simulink model "test_8m_0508"  (R2024a)
settings: Solver=FixedStepAuto  StartTime=0.0  StopTime=30  FixedStep=dt  RelTol=1e-3
values from neighbouring files (symbols this model uses):
  attitude_0 = [0; -90;  -0]    [ini_param_8m_0522.m]
  b = 4.0    (= 4)    [ini_param_8m_0522.m]
  cbar = 0.75    [ini_param_8m_0522.m]
  dt = 0.004    [ini_param_8m_0522.m]
  H = 1000    [ini_param_8m_0522.m]
  N_data = [0,200, 491, 804, 1077, 1344, 1559, 1832, 2078, 2318, 2579,            2864, 3117, 3371, 3608.2, 3872, 4055.7, 4291, 4507, 4739, 4935]'    [cal_motor.m]
  N_pwm = 0.01*[0, 5 ,10 ,15 ,20 ,25 ,30 ,35,40, 45 ,50 ,              55 ,60 ,65 ,70, 75, 80 , 85 ,90 ,95 ,100]'    [cal_motor.m]
  pitch_rate_K = 1    [ini_param_8m_0522.m]
  roll_rate_K = 1    [ini_param_8m_0522.m]
  S = 6.0    (= 6)    [ini_param_8m_0522.m]
  Ts = 0.05    [ini_param_8m_0522.m]
  Ts_sur = 0.25    [ini_param_8m_0522.m]
  yaw_rate_K = 1    [ini_param_8m_0522.m]
undefined symbols (not defined in the file or in its folder): sigbuilder_block, UAV
libraries: slpidlib x9, simulink_extras x6, sharedtransform x2, shared6dof x1
(part 11 of 11)

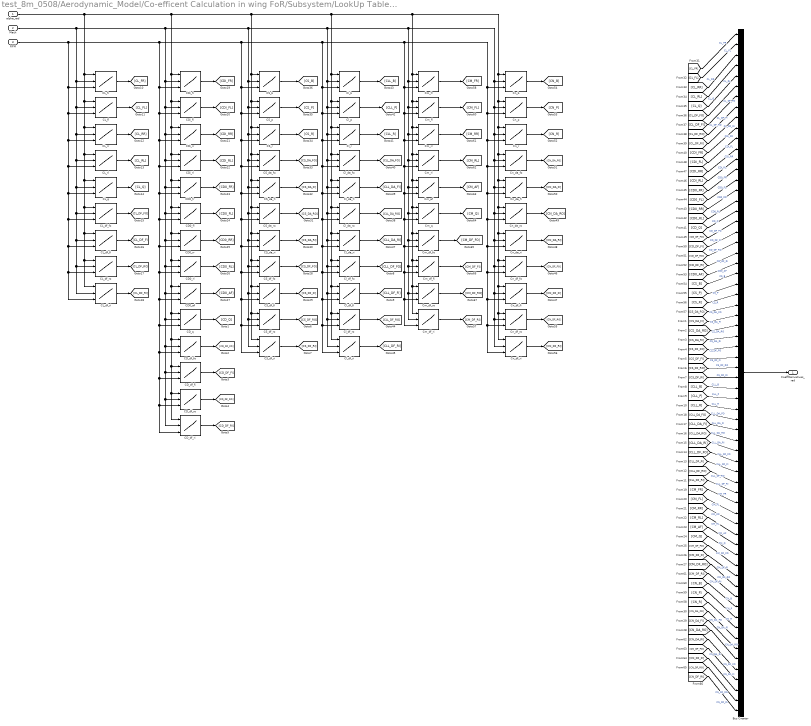
== system test_8m_0508/Aerodynamic_Model/Co-efficent Calculation in wing FoR/Subsystem/LookUp Table for Coeffients_WS8 ==
  alpha_rad : Inport
  Mach : Inport  Port=2
  RPM : Inport  Port=3
  Bus Creator : BusCreator  Inputs=66
  CD0_af : Lookup_n-D  NumberOfTableDimensions=3  DataSpecification=Lookup table object  LookupTableObject=CD0_af  BreakpointsForDimension3=[5, 7]  Table=reshape(repmat([4 5 6;16 19 20;10 18 23],1,2),[3,3,2])  InternalRulePriority=Speed  RndMeth=Simplest
      settings: InputPortMap=u0,u1,u2
  CD0_fl : Lookup_n-D  NumberOfTableDimensions=3  DataSpecification=Lookup table object  LookupTableObject=CD0_fl  BreakpointsForDimension3=[5, 7]  Table=reshape(repmat([4 5 6;16 19 20;10 18 23],1,2),[3,3,2])  InternalRulePriority=Speed  RndMeth=Simplest
      settings: InputPortMap=u0,u1,u2
  CD0_fr : Lookup_n-D  NumberOfTableDimensions=3  DataSpecification=Lookup table object  LookupTableObject=CD0_fr  BreakpointsForDimension3=[5, 7]  Table=reshape(repmat([4 5 6;16 19 20;10 18 23],1,2),[3,3,2])  InternalRulePriority=Speed  RndMeth=Simplest
      settings: InputPortMap=u0,u1,u2
  CD0_rl : Lookup_n-D  NumberOfTableDimensions=3  DataSpecification=Lookup table object  LookupTableObject=CD0_rl  BreakpointsForDimension3=[5, 7]  Table=reshape(repmat([4 5 6;16 19 20;10 18 23],1,2),[3,3,2])  InternalRulePriority=Speed  RndMeth=Simplest
      settings: InputPortMap=u0,u1,u2
  CD0_rr : Lookup_n-D  NumberOfTableDimensions=3  DataSpecification=Lookup table object  LookupTableObject=CD0_rr  BreakpointsForDimension3=[5, 7]  Table=reshape(repmat([4 5 6;16 19 20;10 18 23],1,2),[3,3,2])  InternalRulePriority=Speed  RndMeth=Simplest
      settings: InputPortMap=u0,u1,u2
  CD_df_fi : Lookup_n-D  NumberOfTableDimensions=3  DataSpecification=Lookup table object  LookupTableObject=CD_df_fi  BreakpointsForDimension3=[5, 7]  Table=reshape(repmat([4 5 6;16 19 20;10 18 23],1,2),[3,3,2])  InternalRulePriority=Speed  RndMeth=Simplest
      settings: InputPortMap=u0,u1,u2
  CD_df_fo : Lookup_n-D  NumberOfTableDimensions=3  DataSpecification=Lookup table object  LookupTableObject=CD_df_fo  BreakpointsForDimension3=[5, 7]  Table=reshape(repmat([4 5 6;16 19 20;10 18 23],1,2),[3,3,2])  InternalRulePriority=Speed  RndMeth=Simplest
      settings: InputPortMap=u0,u1,u2
  CD_df_ri : Lookup_n-D  NumberOfTableDimensions=3  DataSpecification=Lookup table object  LookupTableObject=CD_df_ri  BreakpointsForDimension3=[5, 7]  Table=reshape(repmat([4 5 6;16 19 20;10 18 23],1,2),[3,3,2])  InternalRulePriority=Speed  RndMeth=Simplest
      settings: InputPortMap=u0,u1,u2
  CD_df_ro : Lookup_n-D  NumberOfTableDimensions=3  DataSpecification=Lookup table object  LookupTableObject=CD_df_ro  BreakpointsForDimension3=[5, 7]  Table=reshape(repmat([4 5 6;16 19 20;10 18 23],1,2),[3,3,2])  InternalRulePriority=Speed  RndMeth=Simplest
      settings: InputPortMap=u0,u1,u2
  CD_q : Lookup_n-D  NumberOfTableDimensions=3  DataSpecification=Lookup table object  LookupTableObject=CD_q  BreakpointsForDimension3=[5, 7]  Table=reshape(repmat([4 5 6;16 19 20;10 18 23],1,2),[3,3,2])  InternalRulePriority=Speed  RndMeth=Simplest
      settings: InputPortMap=u0,u1,u2
  CDi_fl : Lookup_n-D  NumberOfTableDimensions=3  DataSpecification=Lookup table object  LookupTableObject=CDi_fl  BreakpointsForDimension3=[5, 7]  Table=reshape(repmat([4 5 6;16 19 20;10 18 23],1,2),[3,3,2])  InternalRulePriority=Speed  RndMeth=Simplest
      settings: InputPortMap=u0,u1,u2
  CDi_fr : Lookup_n-D  NumberOfTableDimensions=3  DataSpecification=Lookup table object  LookupTableObject=CDi_fr  BreakpointsForDimension3=[5, 7]  Table=reshape(repmat([4 5 6;16 19 20;10 18 23],1,2),[3,3,2])  InternalRulePriority=Speed  RndMeth=Simplest
      settings: InputPortMap=u0,u1,u2
  CDi_rl : Lookup_n-D  NumberOfTableDimensions=3  DataSpecification=Lookup table object  LookupTableObject=CDi_rl  BreakpointsForDimension3=[5, 7]  Table=reshape(repmat([4 5 6;16 19 20;10 18 23],1,2),[3,3,2])  InternalRulePriority=Speed  RndMeth=Simplest
      settings: InputPortMap=u0,u1,u2
  CDi_rr : Lookup_n-D  NumberOfTableDimensions=3  DataSpecification=Lookup table object  LookupTableObject=CDi_rr  BreakpointsForDimension3=[5, 7]  Table=reshape(repmat([4 5 6;16 19 20;10 18 23],1,2),[3,3,2])  InternalRulePriority=Speed  RndMeth=Simplest
      settings: InputPortMap=u0,u1,u2
  CL_df_fi : Lookup_n-D  NumberOfTableDimensions=3  DataSpecification=Lookup table object  LookupTableObject=CL_df_fi  BreakpointsForDimension3=[5, 7]  Table=reshape(repmat([4 5 6;16 19 20;10 18 23],1,2),[3,3,2])  InternalRulePriority=Speed  RndMeth=Simplest
      settings: InputPortMap=u0,u1,u2
  CL_df_fo : Lookup_n-D  NumberOfTableDimensions=3  DataSpecification=Lookup table object  LookupTableObject=CL_df_fo  BreakpointsForDimension3=[5, 7]  Table=reshape(repmat([4 5 6;16 19 20;10 18 23],1,2),[3,3,2])  InternalRulePriority=Speed  RndMeth=Simplest
      settings: InputPortMap=u0,u1,u2
  CL_df_ri : Lookup_n-D  NumberOfTableDimensions=3  DataSpecification=Lookup table object  LookupTableObject=CL_df_ri  BreakpointsForDimension3=[5, 7]  Table=reshape(repmat([4 5 6;16 19 20;10 18 23],1,2),[3,3,2])  InternalRulePriority=Speed  RndMeth=Simplest
      settings: InputPortMap=u0,u1,u2
  CL_df_ro : Lookup_n-D  NumberOfTableDimensions=3  DataSpecification=Lookup table object  LookupTableObject=CL_df_ro  BreakpointsForDimension3=[5, 7]  Table=reshape(repmat([4 5 6;16 19 20;10 18 23],1,2),[3,3,2])  InternalRulePriority=Speed  RndMeth=Simplest
      settings: InputPortMap=u0,u1,u2
  CL_fl : Lookup_n-D  NumberOfTableDimensions=3  DataSpecification=Lookup table object  LookupTableObject=CL_fl  BreakpointsForDimension3=[5, 7]  Table=reshape(repmat([4 5 6;16 19 20;10 18 23],1,2),[3,3,2])  InternalRulePriority=Speed  RndMeth=Simplest
      settings: InputPortMap=u0,u1,u2
  CL_fr : Lookup_n-D  NumberOfTableDimensions=3  DataSpecification=Lookup table object  LookupTableObject=CL_fr  BreakpointsForDimension3=[5, 7]  Table=reshape(repmat([4 5 6;16 19 20;10 18 23],1,2),[3,3,2])  InternalRulePriority=Speed  RndMeth=Simplest
      settings: InputPortMap=u0,u1,u2
  CL_q : Lookup_n-D  NumberOfTableDimensions=3  DataSpecification=Lookup table object  LookupTableObject=CL_q  BreakpointsForDimension3=[5, 7]  Table=reshape(repmat([4 5 6;16 19 20;10 18 23],1,2),[3,3,2])  InternalRulePriority=Speed  RndMeth=Simplest
      settings: InputPortMap=u0,u1,u2
  CL_rl : Lookup_n-D  NumberOfTableDimensions=3  DataSpecification=Lookup table object  LookupTableObject=CL_rl  BreakpointsForDimension3=[5, 7]  Table=reshape(repmat([4 5 6;16 19 20;10 18 23],1,2),[3,3,2])  InternalRulePriority=Speed  RndMeth=Simplest
      settings: InputPortMap=u0,u1,u2
  CL_rr : Lookup_n-D  NumberOfTableDimensions=3  DataSpecification=Lookup table object  LookupTableObject=CL_rr  BreakpointsForDimension3=[5, 7]  Table=reshape(repmat([4 5 6;16 19 20;10 18 23],1,2),[3,3,2])  InternalRulePriority=Speed  RndMeth=Simplest
      settings: InputPortMap=u0,u1,u2
  CS_b : Lookup_n-D  NumberOfTableDimensions=3  DataSpecification=Lookup table object  LookupTableObject=CS_b  BreakpointsForDimension3=[5, 7]  Table=reshape(repmat([4 5 6;16 19 20;10 18 23],1,2),[3,3,2])  InternalRulePriority=Speed  RndMeth=Simplest
      settings: InputPortMap=u0,u1,u2
  CS_da_fi : Lookup_n-D  NumberOfTableDimensions=3  DataSpecification=Lookup table object  LookupTableObject=CS_da_fi  BreakpointsForDimension3=[5, 7]  Table=reshape(repmat([4 5 6;16 19 20;10 18 23],1,2),[3,3,2])  InternalRulePriority=Speed  RndMeth=Simplest
      settings: InputPortMap=u0,u1,u2
  CS_da_fo : Lookup_n-D  NumberOfTableDimensions=3  DataSpecification=Lookup table object  LookupTableObject=CS_da_fo  BreakpointsForDimension3=[5, 7]  Table=reshape(repmat([4 5 6;16 19 20;10 18 23],1,2),[3,3,2])  InternalRulePriority=Speed  RndMeth=Simplest
      settings: InputPortMap=u0,u1,u2
  CS_da_ri : Lookup_n-D  NumberOfTableDimensions=3  DataSpecification=Lookup table object  LookupTableObject=CS_da_ri  BreakpointsForDimension3=[5, 7]  Table=reshape(repmat([4 5 6;16 19 20;10 18 23],1,2),[3,3,2])  InternalRulePriority=Speed  RndMeth=Simplest
      settings: InputPortMap=u0,u1,u2
  CS_da_ro : Lookup_n-D  NumberOfTableDimensions=3  DataSpecification=Lookup table object  LookupTableObject=CS_da_ro  BreakpointsForDimension3=[5, 7]  Table=reshape(repmat([4 5 6;16 19 20;10 18 23],1,2),[3,3,2])  InternalRulePriority=Speed  RndMeth=Simplest
      settings: InputPortMap=u0,u1,u2
  CS_df_fi : Lookup_n-D  NumberOfTableDimensions=3  DataSpecification=Lookup table object  LookupTableObject=CS_df_fi  BreakpointsForDimension3=[5, 7]  Table=reshape(repmat([4 5 6;16 19 20;10 18 23],1,2),[3,3,2])  InternalRulePriority=Speed  RndMeth=Simplest
      settings: InputPortMap=u0,u1,u2
  CS_df_fo : Lookup_n-D  NumberOfTableDimensions=3  DataSpecification=Lookup table object  LookupTableObject=CS_df_fo  BreakpointsForDimension3=[5, 7]  Table=reshape(repmat([4 5 6;16 19 20;10 18 23],1,2),[3,3,2])  InternalRulePriority=Speed  RndMeth=Simplest
      settings: InputPortMap=u0,u1,u2
  CS_df_ri : Lookup_n-D  NumberOfTableDimensions=3  DataSpecification=Lookup table object  LookupTableObject=CS_df_ri  BreakpointsForDimension3=[5, 7]  Table=reshape(repmat([4 5 6;16 19 20;10 18 23],1,2),[3,3,2])  InternalRulePriority=Speed  RndMeth=Simplest
      settings: InputPortMap=u0,u1,u2
  CS_df_ro : Lookup_n-D  NumberOfTableDimensions=3  DataSpecification=Lookup table object  LookupTableObject=CS_df_ro  BreakpointsForDimension3=[5, 7]  Table=reshape(repmat([4 5 6;16 19 20;10 18 23],1,2),[3,3,2])  InternalRulePriority=Speed  RndMeth=Simplest
      settings: InputPortMap=u0,u1,u2
  CS_p : Lookup_n-D  NumberOfTableDimensions=3  DataSpecification=Lookup table object  LookupTableObject=CS_p  BreakpointsForDimension3=[5, 7]  Table=reshape(repmat([4 5 6;16 19 20;10 18 23],1,2),[3,3,2])  InternalRulePriority=Speed  RndMeth=Simplest
      settings: InputPortMap=u0,u1,u2
  CS_r : Lookup_n-D  NumberOfTableDimensions=3  DataSpecification=Lookup table object  LookupTableObject=CS_r  BreakpointsForDimension3=[5, 7]  Table=reshape(repmat([4 5 6;16 19 20;10 18 23],1,2),[3,3,2])  InternalRulePriority=Speed  RndMeth=Simplest
      settings: InputPortMap=u0,u1,u2
  Cl_b : Lookup_n-D  NumberOfTableDimensions=3  DataSpecification=Lookup table object  LookupTableObject=Cl_b  BreakpointsForDimension3=[5, 7]  Table=reshape(repmat([4 5 6;16 19 20;10 18 23],1,2),[3,3,2])  InternalRulePriority=Speed  RndMeth=Simplest
      settings: InputPortMap=u0,u1,u2
  Cl_da_fi : Lookup_n-D  NumberOfTableDimensions=3  DataSpecification=Lookup table object  LookupTableObject=Cl_da_fi  BreakpointsForDimension3=[5, 7]  Table=reshape(repmat([4 5 6;16 19 20;10 18 23],1,2),[3,3,2])  InternalRulePriority=Speed  RndMeth=Simplest
      settings: InputPortMap=u0,u1,u2
  Cl_da_fo : Lookup_n-D  NumberOfTableDimensions=3  DataSpecification=Lookup table object  LookupTableObject=Cl_da_fo  BreakpointsForDimension3=[5, 7]  Table=reshape(repmat([4 5 6;16 19 20;10 18 23],1,2),[3,3,2])  InternalRulePriority=Speed  RndMeth=Simplest
      settings: InputPortMap=u0,u1,u2
  Cl_da_ri : Lookup_n-D  NumberOfTableDimensions=3  DataSpecification=Lookup table object  LookupTableObject=Cl_da_ri  BreakpointsForDimension3=[5, 7]  Table=reshape(repmat([4 5 6;16 19 20;10 18 23],1,2),[3,3,2])  InternalRulePriority=Speed  RndMeth=Simplest
      settings: InputPortMap=u0,u1,u2
  Cl_da_ro : Lookup_n-D  NumberOfTableDimensions=3  DataSpecification=Lookup table object  LookupTableObject=Cl_da_ro  BreakpointsForDimension3=[5, 7]  Table=reshape(repmat([4 5 6;16 19 20;10 18 23],1,2),[3,3,2])  InternalRulePriority=Speed  RndMeth=Simplest
      settings: InputPortMap=u0,u1,u2
  Cl_df_fi : Lookup_n-D  NumberOfTableDimensions=3  DataSpecification=Lookup table object  LookupTableObject=Cl_df_fi  BreakpointsForDimension3=[5, 7]  Table=reshape(repmat([4 5 6;16 19 20;10 18 23],1,2),[3,3,2])  InternalRulePriority=Speed  RndMeth=Simplest
      settings: InputPortMap=u0,u1,u2
  Cl_df_fo : Lookup_n-D  NumberOfTableDimensions=3  DataSpecification=Lookup table object  LookupTableObject=Cl_df_fo  BreakpointsForDimension3=[5, 7]  Table=reshape(repmat([4 5 6;16 19 20;10 18 23],1,2),[3,3,2])  InternalRulePriority=Speed  RndMeth=Simplest
      settings: InputPortMap=u0,u1,u2
  Cl_df_ri : Lookup_n-D  NumberOfTableDimensions=3  DataSpecification=Lookup table object  LookupTableObject=Cl_df_ri  BreakpointsForDimension3=[5, 7]  Table=reshape(repmat([4 5 6;16 19 20;10 18 23],1,2),[3,3,2])  InternalRulePriority=Speed  RndMeth=Simplest
      settings: InputPortMap=u0,u1,u2
  Cl_df_ro : Lookup_n-D  NumberOfTableDimensions=3  DataSpecification=Lookup table object  LookupTableObject=Cl_df_ro  BreakpointsForDimension3=[5, 7]  Table=reshape(repmat([4 5 6;16 19 20;10 18 23],1,2),[3,3,2])  InternalRulePriority=Speed  RndMeth=Simplest
      settings: InputPortMap=u0,u1,u2
  Cl_p : Lookup_n-D  NumberOfTableDimensions=3  DataSpecification=Lookup table object  LookupTableObject=Cl_p  BreakpointsForDimension3=[5, 7]  Table=reshape(repmat([4 5 6;16 19 20;10 18 23],1,2),[3,3,2])  InternalRulePriority=Speed  RndMeth=Simplest
      settings: InputPortMap=u0,u1,u2
  Cl_r : Lookup_n-D  NumberOfTableDimensions=3  DataSpecification=Lookup table object  LookupTableObject=Cl_r  BreakpointsForDimension3=[5, 7]  Table=reshape(repmat([4 5 6;16 19 20;10 18 23],1,2),[3,3,2])  InternalRulePriority=Speed  RndMeth=Simplest
      settings: InputPortMap=u0,u1,u2
  Cm_af : Lookup_n-D  NumberOfTableDimensions=3  DataSpecification=Lookup table object  LookupTableObject=Cm_af  BreakpointsForDimension3=[5, 7]  Table=reshape(repmat([4 5 6;16 19 20;10 18 23],1,2),[3,3,2])  InternalRulePriority=Speed  RndMeth=Simplest
      settings: InputPortMap=u0,u1,u2
  Cm_df_fi : Lookup_n-D  NumberOfTableDimensions=3  DataSpecification=Lookup table object  LookupTableObject=Cm_df_fi  BreakpointsForDimension3=[5, 7]  Table=reshape(repmat([4 5 6;16 19 20;10 18 23],1,2),[3,3,2])  InternalRulePriority=Speed  RndMeth=Simplest
      settings: InputPortMap=u0,u1,u2
  Cm_df_fo : Lookup_n-D  NumberOfTableDimensions=3  DataSpecification=Lookup table object  LookupTableObject=Cm_df_fo  BreakpointsForDimension3=[5, 7]  Table=reshape(repmat([4 5 6;16 19 20;10 18 23],1,2),[3,3,2])  InternalRulePriority=Speed  RndMeth=Simplest
      settings: InputPortMap=u0,u1,u2
  Cm_df_ri : Lookup_n-D  NumberOfTableDimensions=3  DataSpecification=Lookup table object  LookupTableObject=Cm_df_ri  BreakpointsForDimension3=[5, 7]  Table=reshape(repmat([4 5 6;16 19 20;10 18 23],1,2),[3,3,2])  InternalRulePriority=Speed  RndMeth=Simplest
      settings: InputPortMap=u0,u1,u2
  Cm_df_ro : Lookup_n-D  NumberOfTableDimensions=3  DataSpecification=Lookup table object  LookupTableObject=Cm_df_ro  BreakpointsForDimension3=[5, 7]  Table=reshape(repmat([4 5 6;16 19 20;10 18 23],1,2),[3,3,2])  InternalRulePriority=Speed  RndMeth=Simplest
      settings: InputPortMap=u0,u1,u2
  Cm_fl : Lookup_n-D  NumberOfTableDimensions=3  DataSpecification=Lookup table object  LookupTableObject=Cm_fl  BreakpointsForDimension3=[5, 7]  Table=reshape(repmat([4 5 6;16 19 20;10 18 23],1,2),[3,3,2])  InternalRulePriority=Speed  RndMeth=Simplest
      settings: InputPortMap=u0,u1,u2
  Cm_fr : Lookup_n-D  NumberOfTableDimensions=3  DataSpecification=Lookup table object  LookupTableObject=Cm_fr  BreakpointsForDimension3=[5, 7]  Table=reshape(repmat([4 5 6;16 19 20;10 18 23],1,2),[3,3,2])  InternalRulePriority=Speed  RndMeth=Simplest
      settings: InputPortMap=u0,u1,u2
  Cm_q : Lookup_n-D  NumberOfTableDimensions=3  DataSpecification=Lookup table object  LookupTableObject=Cm_q  BreakpointsForDimension3=[5, 7]  Table=reshape(repmat([4 5 6;16 19 20;10 18 23],1,2),[3,3,2])  InternalRulePriority=Speed  RndMeth=Simplest
      settings: InputPortMap=u0,u1,u2
  Cm_rl : Lookup_n-D  NumberOfTableDimensions=3  DataSpecification=Lookup table object  LookupTableObject=Cm_rl  BreakpointsForDimension3=[5, 7]  Table=reshape(repmat([4 5 6;16 19 20;10 18 23],1,2),[3,3,2])  InternalRulePriority=Speed  RndMeth=Simplest
      settings: InputPortMap=u0,u1,u2
  Cm_rr : Lookup_n-D  NumberOfTableDimensions=3  DataSpecification=Lookup table object  LookupTableObject=Cm_rr  BreakpointsForDimension3=[5, 7]  Table=reshape(repmat([4 5 6;16 19 20;10 18 23],1,2),[3,3,2])  InternalRulePriority=Speed  RndMeth=Simplest
      settings: InputPortMap=u0,u1,u2
  Cn_b : Lookup_n-D  NumberOfTableDimensions=3  DataSpecification=Lookup table object  LookupTableObject=Cn_b  BreakpointsForDimension3=[5, 7]  Table=reshape(repmat([4 5 6;16 19 20;10 18 23],1,2),[3,3,2])  InternalRulePriority=Speed  RndMeth=Simplest
      settings: InputPortMap=u0,u1,u2
  Cn_da_fi : Lookup_n-D  NumberOfTableDimensions=3  DataSpecification=Lookup table object  LookupTableObject=Cn_da_fi  BreakpointsForDimension3=[5, 7]  Table=reshape(repmat([4 5 6;16 19 20;10 18 23],1,2),[3,3,2])  InternalRulePriority=Speed  RndMeth=Simplest
      settings: InputPortMap=u0,u1,u2
  Cn_da_fo : Lookup_n-D  NumberOfTableDimensions=3  DataSpecification=Lookup table object  LookupTableObject=Cn_da_fo  BreakpointsForDimension3=[5, 7]  Table=reshape(repmat([4 5 6;16 19 20;10 18 23],1,2),[3,3,2])  InternalRulePriority=Speed  RndMeth=Simplest
      settings: InputPortMap=u0,u1,u2
  Cn_da_ri : Lookup_n-D  NumberOfTableDimensions=3  DataSpecification=Lookup table object  LookupTableObject=Cn_da_ri  BreakpointsForDimension3=[5, 7]  Table=reshape(repmat([4 5 6;16 19 20;10 18 23],1,2),[3,3,2])  InternalRulePriority=Speed  RndMeth=Simplest
      settings: InputPortMap=u0,u1,u2
  Cn_da_ro : Lookup_n-D  NumberOfTableDimensions=3  DataSpecification=Lookup table object  LookupTableObject=Cn_da_ro  BreakpointsForDimension3=[5, 7]  Table=reshape(repmat([4 5 6;16 19 20;10 18 23],1,2),[3,3,2])  InternalRulePriority=Speed  RndMeth=Simplest
      settings: InputPortMap=u0,u1,u2
  Cn_df_fi : Lookup_n-D  NumberOfTableDimensions=3  DataSpecification=Lookup table object  LookupTableObject=Cn_df_fi  BreakpointsForDimension3=[5, 7]  Table=reshape(repmat([4 5 6;16 19 20;10 18 23],1,2),[3,3,2])  InternalRulePriority=Speed  RndMeth=Simplest
      settings: InputPortMap=u0,u1,u2
  Cn_df_fo : Lookup_n-D  NumberOfTableDimensions=3  DataSpecification=Lookup table object  LookupTableObject=Cn_df_fo  BreakpointsForDimension3=[5, 7]  Table=reshape(repmat([4 5 6;16 19 20;10 18 23],1,2),[3,3,2])  InternalRulePriority=Speed  RndMeth=Simplest
      settings: InputPortMap=u0,u1,u2
  Cn_df_ri : Lookup_n-D  NumberOfTableDimensions=3  DataSpecification=Lookup table object  LookupTableObject=Cn_df_ri  BreakpointsForDimension3=[5, 7]  Table=reshape(repmat([4 5 6;16 19 20;10 18 23],1,2),[3,3,2])  InternalRulePriority=Speed  RndMeth=Simplest
      settings: InputPortMap=u0,u1,u2
  Cn_df_ro : Lookup_n-D  NumberOfTableDimensions=3  DataSpecification=Lookup table object  LookupTableObject=Cn_df_ro  BreakpointsForDimension3=[5, 7]  Table=reshape(repmat([4 5 6;16 19 20;10 18 23],1,2),[3,3,2])  InternalRulePriority=Speed  RndMeth=Simplest
      settings: InputPortMap=u0,u1,u2
  Cn_p : Lookup_n-D  NumberOfTableDimensions=3  DataSpecification=Lookup table object  LookupTableObject=Cn_p  BreakpointsForDimension3=[5, 7]  Table=reshape(repmat([4 5 6;16 19 20;10 18 23],1,2),[3,3,2])  InternalRulePriority=Speed  RndMeth=Simplest
      settings: InputPortMap=u0,u1,u2
  Cn_r : Lookup_n-D  NumberOfTableDimensions=3  DataSpecification=Lookup table object  LookupTableObject=Cn_r  BreakpointsForDimension3=[5, 7]  Table=reshape(repmat([4 5 6;16 19 20;10 18 23],1,2),[3,3,2])  InternalRulePriority=Speed  RndMeth=Simplest
      settings: InputPortMap=u0,u1,u2
  CoeffDerivatives_rad : Outport
  wires:
  Bus Creator/1 -> CoeffDerivatives_rad/1
  [CD_DF_FO] -> Bus Creator/19  "CD_DF_FO"
  [CL_Q] -> Bus Creator/5  "CL_Q"
  [CL_RL] -> Bus Creator/4  "CL_RL"
  [CS_B] -> Bus Creator/24  "CS_B"
  [CD0_AF] -> Bus Creator/23  "CD0_AF"
  [CD_DF_FI] -> Bus Creator/20  "CD_DF_FI"
  [CD_Q] -> Bus Creator/18  "CD_Q"
  [CDI_FL] -> Bus Creator/11  "CDI_FL"
  [CL_DF_RI] -> Bus Creator/9  "CL_DF_RI"
  [CD0_FL] -> Bus Creator/15  "CD0_FL"
  [CD0_RL] -> Bus Creator/17  "CD0_RL"
  [CL_FR] -> Bus Creator/1  "CL_FR"
  [CD0_FR] -> Bus Creator/14  "CD0_FR"
  [CDI_FR] -> Bus Creator/10  "CDI_FR"
  [CDI_RL] -> Bus Creator/13  "CDI_RL"
  [CS_R] -> Bus Creator/26  "CS_R"
  [CDI_RR] -> Bus Creator/12  "CDI_RR"
  [CL_RR] -> Bus Creator/3  "CL_RR"
  [CL_DF_FI] -> Bus Creator/7  "CL_DF_FI"
  [CD_DF_RO] -> Bus Creator/21  "CD_DF_RO"
  [CD_DF_RI] -> Bus Creator/22  "CD_DF_RI"
  [CL_DF_FO] -> Bus Creator/6  "CL_DF_FO"
  [CS_DA_FO] -> Bus Creator/27  "CS_DA_FO"
  [CD0_RR] -> Bus Creator/16  "CD0_RR"
  [CS_P] -> Bus Creator/25  "CS_P"
  [CL_DF_RO] -> Bus Creator/8  "CL_DF_RO"
  [CL_FL] -> Bus Creator/2  "CL_FL"
  CL_fr/1 -> [CL_FR]
  CL_fl/1 -> [CL_FL]
  CL_rr/1 -> [CL_RR]
  CL_rl/1 -> [CL_RL]
  CL_q/1 -> [CL_Q]
  CL_df_fo/1 -> [CL_DF_FO]
  CL_df_fi/1 -> [CL_DF_FI]
  CL_df_ro/1 -> [CL_DF_RO]
  CL_df_ri/1 -> [CL_DF_RI]
  CDi_fr/1 -> [CDI_FR]
  CDi_fl/1 -> [CDI_FL]
  CDi_rr/1 -> [CDI_RR]
  CDi_rl/1 -> [CDI_RL]
  CD0_fr/1 -> [CD0_FR]
  CD0_fl/1 -> [CD0_FL]
  CD0_rr/1 -> [CD0_RR]
  CD0_rl/1 -> [CD0_RL]
  CD0_af/1 -> [CD0_AF]
  CD_q/1 -> [CD_Q]
  CD_df_fo/1 -> [CD_DF_FO]
  CD_df_fi/1 -> [CD_DF_FI]
  CS_b/1 -> [CS_B]
  CS_p/1 -> [CS_P]
  CS_r/1 -> [CS_R]
  CS_da_fo/1 -> [CS_DA_FO]
  CS_da_fi/1 -> [CS_DA_FI]
  CS_da_ro/1 -> [CS_DA_RO]
  CS_da_ri/1 -> [CS_DA_RI]
  CS_df_fo/1 -> [CS_DF_FO]
  CS_df_fi/1 -> [CS_DF_FI]
  CS_df_ro/1 -> [CS_DF_RO]
  CS_df_ri/1 -> [CS_DF_RI]
  Cl_b/1 -> [CLL_B]
  Cl_p/1 -> [CLL_P]
  Cl_r/1 -> [CLL_R]
  Cl_da_fo/1 -> [CLL_DA_FO]
  Cl_da_fi/1 -> [CLL_DA_FI]
  Cl_da_ro/1 -> [CLL_DA_RO]
  Cl_da_ri/1 -> [CLL_DA_RI]
  Cl_df_fo/1 -> [CLL_DF_FO]
  Cl_df_fi/1 -> [CLL_DF_FI]
  Cl_df_ro/1 -> [CLL_DF_RO]
  Cl_df_ri/1 -> [CLL_DF_RI]
  Cm_fr/1 -> [CM_FR]
  Cm_fl/1 -> [CM_FL]
  Cm_rr/1 -> [CM_RR]
  Cm_rl/1 -> [CM_RL]
  Cm_af/1 -> [CM_AF]
  Cm_q/1 -> [CM_Q]
  Cm_df_fo/1 -> [CM_DF_FO]
  Cm_df_fi/1 -> [CM_DF_FI]
  Cm_df_ro/1 -> [CM_DF_RO]
  Cm_df_ri/1 -> [CM_DF_RI]
  Cn_b/1 -> [CN_B]
  Cn_p/1 -> [CN_P]
  Cn_r/1 -> [CN_R]
  Cn_da_fo/1 -> [CN_DA_FO]
  Cn_da_fi/1 -> [CN_DA_FI]
  Cn_da_ro/1 -> [CN_DA_RO]
  Cn_da_ri/1 -> [CN_DA_RI]
  Cn_df_fo/1 -> [CN_DF_FO]
  Cn_df_fi/1 -> [CN_DF_FI]
  Cn_df_ro/1 -> [CN_DF_RO]
  Cn_df_ri/1 -> [CN_DF_RI]
  CD_df_ro/1 -> [CD_DF_RO]
  CD_df_ri/1 -> [CD_DF_RI]
  alpha_rad/1 -> CL_df_ri/1, CL_df_ro/1, CL_df_fi/1, CL_df_fo/1, CL_q/1, CL_rl/1, CL_rr/1, CL_fl/1, CL_fr/1, CS_df_ri/1, CS_df_ro/1, CS_df_fi/1, CS_df_fo/1, CS_da_ri/1, CS_da_ro/1, CS_da_fi/1, CS_da_fo/1, CS_r/1, CS_p/1, CS_b/1, Cl_df_ri/1, Cl_df_ro/1, Cl_df_fi/1, Cl_df_fo/1, Cl_da_ri/1, Cl_da_ro/1, Cl_da_fi/1, Cl_da_fo/1, Cl_r/1, Cl_p/1, Cl_b/1, Cn_df_ri/1, Cn_df_ro/1, Cn_df_fi/1, Cn_df_fo/1, Cn_da_ri/1, Cn_da_ro/1, Cn_da_fi/1, Cn_da_fo/1, Cn_r/1, Cn_p/1, Cn_b/1, Cm_df_ri/1, Cm_df_ro/1, Cm_df_fi/1, Cm_df_fo/1, Cm_q/1, Cm_af/1, Cm_rl/1, Cm_rr/1, Cm_fl/1, Cm_fr/1, CD_df_ri/1, CD_df_ro/1, CD_df_fi/1, CD_df_fo/1, CD_q/1, CD0_af/1, CD0_rl/1, CD0_rr/1, CD0_fl/1, CD0_fr/1, CDi_rl/1, CDi_rr/1, CDi_fl/1, CDi_fr/1
  Mach/1 -> CL_df_ri/2, CL_df_ro/2, CL_df_fi/2, CL_df_fo/2, CL_q/2, CL_rl/2, CL_rr/2, CL_fl/2, CL_fr/2, Cn_df_ri/2, Cn_df_ro/2, Cn_df_fi/2, Cn_df_fo/2, Cn_da_ri/2, Cn_da_ro/2, Cn_da_fi/2, Cn_da_fo/2, Cn_r/2, Cn_p/2, Cn_b/2, Cm_df_ri/2, Cm_df_ro/2, Cm_df_fi/2, Cm_df_fo/2, Cm_q/2, Cm_af/2, Cm_rl/2, Cm_rr/2, Cm_fl/2, Cm_fr/2, Cl_df_ri/2, Cl_df_ro/2, Cl_df_fi/2, Cl_df_fo/2, Cl_da_ri/2, Cl_da_ro/2, Cl_da_fi/2, Cl_da_fo/2, Cl_r/2, Cl_p/2, Cl_b/2, CS_df_ri/2, CS_df_ro/2, CS_df_fi/2, CS_df_fo/2, CS_da_ri/2, CS_da_ro/2, CS_da_fi/2, CS_da_fo/2, CS_r/2, CS_p/2, CS_b/2, CD_df_ri/2, CD_df_ro/2, CD_df_fi/2, CD_df_fo/2, CD_q/2, CD0_af/2, CD0_rl/2, CD0_rr/2, CD0_fl/2, CD0_fr/2, CDi_rl/2, CDi_rr/2, CDi_fl/2, CDi_fr/2
  RPM/1 -> Cn_da_ro/3, Cn_df_ri/3, Cn_df_ro/3, Cn_df_fi/3, Cn_df_fo/3, Cn_da_ri/3, Cn_da_fi/3, Cn_da_fo/3, Cn_r/3, Cn_p/3, Cn_b/3, Cm_df_ri/3, Cm_df_ro/3, Cm_df_fi/3, Cm_df_fo/3, Cm_q/3, Cm_af/3, Cm_rl/3, Cm_rr/3, Cm_fl/3, Cm_fr/3, Cl_df_ri/3, Cl_df_ro/3, Cl_df_fi/3, Cl_df_fo/3, Cl_da_ri/3, Cl_da_ro/3, Cl_da_fi/3, Cl_da_fo/3, Cl_r/3, Cl_p/3, Cl_b/3, CS_df_ri/3, CS_df_ro/3, CS_df_fi/3, CS_df_fo/3, CS_da_ri/3, CS_da_ro/3, CS_da_fi/3, CS_da_fo/3, CS_r/3, CS_p/3, CS_b/3, CD_df_ri/3, CD_df_ro/3, CD_df_fi/3, CD_df_fo/3, CD_q/3, CD0_af/3, CD0_rl/3, CD0_rr/3, CD0_fl/3, CD0_fr/3, CDi_rl/3, CDi_rr/3, CDi_fl/3, CDi_fr/3, CL_df_ri/3, CL_df_ro/3, CL_df_fi/3, CL_df_fo/3, CL_q/3, CL_rl/3, CL_rr/3, CL_fl/3, CL_fr/3
  [CS_DA_FI] -> Bus Creator/28  "CS_DA_FI"
  [CS_DA_RO] -> Bus Creator/29  "CS_DA_RO"
  [CS_DA_RI] -> Bus Creator/30  "CS_DA_RI"
  [CS_DF_FO] -> Bus Creator/31  "CS_DF_FO"
  [CS_DF_FI] -> Bus Creator/32  "CS_DF_FI"
  [CS_DF_RO] -> Bus Creator/33  "CS_DF_RO"
  [CS_DF_RI] -> Bus Creator/34  "CS_DF_RI"
  [CLL_B] -> Bus Creator/35  "CLL_B"
  [CLL_P] -> Bus Creator/36  "CLL_P"
  [CLL_R] -> Bus Creator/37  "CLL_R"
  [CLL_DA_FO] -> Bus Creator/38  "CLL_DA_FO"
  [CLL_DA_FI] -> Bus Creator/39  "CLL_DA_FI"
  [CLL_DA_RO] -> Bus Creator/40  "CLL_DA_RO"
  [CLL_DA_RI] -> Bus Creator/41  "CLL_DA_RI"
  [CLL_DF_FO] -> Bus Creator/42  "CLL_DF_FO"
  [CLL_DF_FI] -> Bus Creator/43  "CLL_DF_FI"
  [CLL_DF_RO] -> Bus Creator/44  "CLL_DF_RO"
  [CLL_DF_RI] -> Bus Creator/45  "CLL_DF_RI"
  [CM_FR] -> Bus Creator/46  "CM_FR"
  [CM_FL] -> Bus Creator/47  "CM_FL"
  [CM_RR] -> Bus Creator/48  "CM_RR"
  [CM_RL] -> Bus Creator/49  "CM_RL"
  [CM_AF] -> Bus Creator/50  "CM_AF"
  [CM_Q] -> Bus Creator/51  "CM_Q"
  [CM_DF_FO] -> Bus Creator/52  "CM_DF_FO"
  [CM_DF_FI] -> Bus Creator/53  "CM_DF_FI"
  [CM_DF_RO] -> Bus Creator/54  "CM_DF_RO"
  [CM_DF_RI] -> Bus Creator/55  "CM_DF_RI"
  [CN_B] -> Bus Creator/56  "CN_B"
  [CN_P] -> Bus Creator/57  "CN_P"
  [CN_R] -> Bus Creator/58  "CN_R"
  [CN_DA_FO] -> Bus Creator/59  "CN_DA_FO"
  [CN_DA_FI] -> Bus Creator/60  "CN_DA_FI"
  [CN_DA_RO] -> Bus Creator/61  "CN_DA_RO"
  [CN_DA_RI] -> Bus Creator/62  "CN_DA_RI"
  [CN_DF_FO] -> Bus Creator/63  "CN_DF_FO"
  [CN_DF_FI] -> Bus Creator/64  "CN_DF_FI"
  [CN_DF_RO] -> Bus Creator/65  "CN_DF_RO"
  [CN_DF_RI] -> Bus Creator/66  "CN_DF_RI"

== matlab function test_8m_0508/速度控制/速度→加速度 需加限幅/MATLAB Function ==
  data: u1 input; y output; u2 input; u3 input
function y = fcn(u1,u2,u3)
y = zeros(3,1);
y(1)=u1;y(2)=u2;y(3)=u3;

== matlab function test_8m_0508/Environment Function ==
  data: PosEarth input; DensityAir output; AccGravity output
function [DensityAir, AccGravity] = CalculateEnvironment(PosEarth)
%% 1. Sea level standard value
T0 = 288.15;            
rho0 = 1.225;           
g0 = 9.80665;          
R = 287.0528;         
L = 0.0065;             
Re = 6371000;         

%% 2. Protection procedure
Altitude = -PosEarth(3);
if Altitude < 0
    Altitude = 0;
end

%% 3. Gravity acceleration calculation (attenuation with height)
AccGravity = g0 * (Re / (Re + Altitude))^2;

%% 4. Air density calculation (ISA model)
%The atmosphere is divided into troposphere (0~11000m) 
% and lower stratosphere (11000~20000m)

if Altitude < 11000
    T = T0 - L * Altitude;
    Exponent = (g0 / (L * R)) - 1;
    DensityAir = rho0 * (T / T0)^Exponent;
else
    T_strat = 216.65;
    p_11k = 101325 * (T_strat / T0)^(g0 / (L * R));
    p_strat = p_11k * exp(-g0 * (Altitude - 11000) / (R * T_strat));
    DensityAir = p_strat / (R * T_strat);
end

end

== matlab function test_8m_0508/速度控制/角速度环PID 需加限幅/MATLAB Function ==
  data: u1 input; y output; u2 input; u3 input
function y = fcn(u1,u2,u3)
y = zeros(3,1);
y(1)=u1;
y(2)=u2;
y(3)=u3;

== matlab function test_8m_0508/速度控制/Alt2q/XYZ-ZYX ==
  data: u input; y output
function y = fcn(u)
    TEMP =  u;
    y = [TEMP(3);TEMP(2);TEMP(1)];
end

== matlab function test_8m_0508/速度控制/MATLAB Function3 ==
  data: a_des input; q_des output; psi_des input; euler_des output; AccGravity input; StructAircraft parameter; thrust_acc output
function [q_des, euler_des, thrust_acc] = mapAccelerationToAttitude(a_des, psi_des, AccGravity, StructAircraft)
    % 输入:
    % a_des: 期望加速度 3x1 向量 (NED坐标系, m/s^2)
    % psi_des: 期望偏航角 (rad)
    % hover_throttle: 标定的悬停油门值 (0~1)
    
    % 常量定义
    g = AccGravity;
    g_vec = [0; 0; g]; % NED重力向量

   
    % 1. 抵消重力，计算所需的比力向量
    f_des = a_des - g_vec; 
    
    % 2. 计算基准油门
    thrust_acc = norm(f_des);   
    
    % 3. 构建推力坐标系 (Thrust Frame)
    if thrust_acc < 1e-4
        z_T = [0; 0; -1]; % 奇异点保护：如果处于零重力自由落体，默认推力向上
    else
        z_T = -f_des / thrust_acc; 
    end
    % 根据期望 Yaw 构造辅助向量
    x_yaw = [cos(psi_des); sin(psi_des); 0];
    % 机体 Y 轴 (z_T 叉乘 x_yaw)
    y_T = cross(z_T, x_yaw);
    
    if norm(y_T) < 1e-4
        y_T = [0; 1; 0]; % 奇异点保护：如果推力完全水平且和偏航共线
    else
        y_T = y_T / norm(y_T);
    end
    
    x_T = cross(y_T, z_T);
    
    % 推力系到世界系的旋转矩阵
    % “推力坐标系”是飞控外环计算出来的**绝对参考基准**。
    R_W_T = [x_T, y_T, z_T];
    
    % 4. X度安装偏角补偿 (Thrust -> Body)
    % 机身在推力系基础上上仰X度 (绕Y轴旋转)

    theta_offset = (90 - StructAircraft.TiltXd)*pi/180; 
    R_T_B =  euler2rotm_zyx([0;theta_offset;0]);
    % R_T_B = [cos(theta_offset),  0, sin(theta_offset);
    %          0,                  1,                 0;
    %         -sin(theta_offset),  0, cos(theta_offset)];
            
    % 计算最终机体到世界系的旋转矩阵
    R_W_B = R_W_T * R_T_B;
    
    % 5. 旋转矩阵转四元数 [w, x, y, z] (直接写出算法方便你移植C++)
    
    % R_W_B = euler2rotm_zyx(attitude_ref);

    [q_des,euler_des] = rotm2quat_custom(R_W_B);
end
%%
% 辅助函数：旋转矩阵转四元数 (避免依赖 MATLAB 机器人工具箱)
function [q, euler_target] = rotm2quat_custom(R)
    tr = trace(R);
    if tr > 0
        S = sqrt(tr + 1.0) * 2;
        qw = 0.25 * S;
        qx = (R(3,2) - R(2,3)) / S;
        qy = (R(1,3) - R(3,1)) / S;
        qz = (R(2,1) - R(1,2)) / S;
    elseif (R(1,1) > R(2,2)) && (R(1,1) > R(3,3))
        S = sqrt(1.0 + R(1,1) - R(2,2) - R(3,3)) * 2;
        qw = (R(3,2) - R(2,3)) / S;
        qx = 0.25 * S;
        qy = (R(1,2) + R(2,1)) / S;
        qz = (R(1,3) + R(3,1)) / S;
    elseif R(2,2) > R(3,3)
        S = sqrt(1.0 + R(2,2) - R(1,1) - R(3,3)) * 2;
        qw = (R(1,3) - R(3,1)) / S;
        qx = (R(1,2) + R(2,1)) / S;
        qy = 0.25 * S;
        qz = (R(2,3) + R(3,2)) / S;
    else
        S = sqrt(1.0 + R(3,3) - R(1,1) - R(2,2)) * 2;
        qw = (R(2,1) - R(1,2)) / S;
        qx = (R(1,3) + R(3,1)) / S;
        qy = (R(2,3) + R(3,2)) / S;
        qz = 0.25 * S;
    end
    q = [qw, qx, qy, qz];
    q = q / norm(q); % 归一化

    % --- 5. 旋转矩阵转欧拉角 (ZYX顺序，仅用于观测) ---
    % roll (phi), pitch (theta), yaw (psi)
    pitch_obs = asin(-R(3,1));
    roll_obs  = atan2(R(3,2), R(3,3));
    yaw_obs   = atan2(R(2,1), R(1,1));
    
    % 转换为度数输出，方便你直观检查
    euler_target = rad2deg([roll_obs, pitch_obs, yaw_obs]);
end
%%
function R = euler2rotm_zyx(euler)
% euler = [roll; pitch; yaw]  (单位：rad)
% 输出 R 为 3x3 旋转矩阵
% ZYX 顺序：R = Rz(yaw) * Ry(pitch) * Rx(roll)

    phi   = euler(1);   % roll
    theta = euler(2);   % pitch
    psi   = euler(3);   % yaw
    
    % 各角三角函数
    cphi = cos(phi);   sphi = sin(phi);
    cth  = cos(theta); sth  = sin(theta);
    cpsi = cos(psi);   spsi = sin(psi);
    
    % 旋转矩阵
    R = [ ...
        cpsi*cth,  cpsi*sth*sphi - spsi*cphi,  cpsi*sth*cphi + spsi*sphi;
        spsi*cth,  spsi*sth*sphi + cpsi*cphi,  spsi*sth*cphi - cpsi*sphi;
        -sth,      cth*sphi,                   cth*cphi ];

end

== matlab function test_8m_0508/速度控制/位置→速度 需加限幅/MATLAB Function ==
  data: u1 input; y output; u2 input; u3 input
function y = fcn(u1,u2,u3)
y = zeros(3,1);
y(1)=u1;y(2)=u2;y(3)=u3;

== matlab function test_8m_0508/Calc_Forces_Moments_A ==
  data: mot_pwn_in1 input; surpwn_in1 input; F_body output; Pos_E input; Vel_E input; attitude input; Omega_B input; M_body output; Stop output; R_be output; AccGravity input; rho input; StructAircraft parameter; F_aero_b output; F_out_ms output
function [F_body, M_body, Stop, R_be, F_aero_b, F_out_ms] = fcn(mot_pwn_in1, surpwn_in1, Pos_E, Vel_E, attitude, Omega_B, AccGravity, rho, StructAircraft)    
    
    % ==========================================================
    % 1. 状态解析与保护机制
    % ==========================================================
    Stop = 0;
    phi_  = attitude(1);
    theta = attitude(2);
    
    % 姿态异常保护
    if abs(theta) > deg2rad(65) || abs(phi_) > deg2rad(65)
        Stop = 999;
    end

    % 运动学转换
    R_be = cal_R_be(attitude);
    V_b = R_be' * Vel_E; % 地速转体轴空速 (假设无风)

    % ==========================================================
    % 2. 各物理模块受力与力矩解算
    % ==========================================================
    
    % A. 重力解算
    mg = StructAircraft.m * AccGravity;
    F_gravity_b = R_be' * [0; 0; mg];
    
    % B. 动力系统解算 (螺旋桨拉力与反扭 - 已向量化优化)
    [F_out, M_out, F_motor, F_sur, torque_mot, torque_sur] = Cal_Motor_Sur( ...
    mot_pwn_in1, surpwn_in1, StructAircraft); %mot_pwn_in1, surpwn_in1
    % temp1 = [torque_mot' torque_sur'];
    % temp2 = sum(temp1);
    % debug1_1 = [temp1;temp2];    
    F_out_ms_temp = [F_motor F_sur];
    F_out_ms_sum = sum(F_out_ms_temp);
    F_out_ms = [F_out_ms_temp;F_out_ms_sum];

    % C. 地面反作用力解算 (起落架/机腹触地模型)
    [F_ground_b, M_gnd, dz_e] = calc_ground_effect(Pos_E, Vel_E, theta, Omega_B, R_be, mg);
    
    % D. 气动力与舵面解算 (机翼升阻力、下洗效应、操纵面)
    % [F_aero_b, M_aero_b] = calc_aerodynamics(V_b, Aileron_Angle, rho, StructAircraft, StructAerodynamic);
    % LD = 7.1169;
    % F_L = sum(F_sur);
    % F_aero_b = 1/LD*F_L*-V_b/norm(V_b);
    F_aero_b = 0;


    % ==========================================================
    % 3. 总输出汇总
    % ==========================================================    
    F_body = F_out + F_ground_b + F_gravity_b + F_aero_b;
    M_body = M_out + M_gnd;

    % 滤除微小计算截断误差
    M_body(abs(M_body) < 1e-6) = 0;
    
    % 调试输出
    % debug31 = R_be * F_body;
    % debug31 = R_be * F_ground_b;
    % debug1 = dz_e;

    
    %% ==========================================================
    % 内部子函数区域
    % ==========================================================

    % ============== 姿态旋转矩阵 ==============
    function R = cal_R_be(att)
        cphi = cos(att(1)); sphi = sin(att(1));
        cth  = cos(att(2)); sth  = sin(att(2));
        cpsi = cos(att(3)); spsi = sin(att(3));
        
        R = [
            cpsi*cth,  cpsi*sth*sphi - spsi*cphi,  cpsi*sth*cphi + spsi*sphi;
            spsi*cth,  spsi*sth*sphi + cpsi*cphi,  spsi*sth*cphi - cpsi*sphi;
            -sth,      cth*sphi,                   cth*cphi
        ];
    end

    % ==============动力组件==============

    % ============== 地面接触解算 ==============
    function [F_g_b, M_g, dz] = calc_ground_effect(Pos, Vel, th, Omega, R_mat, weight)
        R_geom = 0.2517;
        x_arc = 0;      
        z_arc = -0.1746; 
        
        % 寻找接触点几何
        R_g = abs(z_arc);
        dz = Pos(3) + R_g * (1 - cos(th)); 
        
        if dz >= -0.00 % 发生触地
            k_g = 6e2;   % 刚度
            c_g = 6.5e2; % 阻尼
            
            F_dynamic = -k_g * dz - c_g * Vel(3);
            F_z_g = min(0, -weight + F_dynamic); % 地面只能提供向上的支撑力(Z轴负方向)
            
            % 水平摩擦
            mu = 0.5; smooth_factor = 50;
            F_x_g = mu * F_z_g * tanh(smooth_factor * Vel(1));
            F_y_g = mu * F_z_g * tanh(smooth_factor * Vel(2));
            
            F_ground_e = [F_x_g; F_y_g; F_z_g];
            F_g_b = R_mat' * F_ground_e;
            
            % 地面力矩
            r_cp_x = x_arc - R_geom * sin(th);
            r_cp_z = z_arc + R_geom * cos(th);
            M_roll_resist = -0.2 * Omega(2); % 滚动阻尼矩
            M_gnd_y = r_cp_z * F_g_b(1) - r_cp_x * F_g_b(3);
            
            M_g = [0; M_gnd_y + M_roll_resist; 0];
        else
            F_g_b = [0; 0; 0];
            M_g   = [0; 0; 0];
        end
    end

    % ============== 气动力学解算 ==============
    function [F_a_b, M_a_b] = calc_aerodynamics(V_body, Aileron, rho_air, Aircraft, Aero)
        u = V_body(1); v = V_body(2); w = V_body(3);
        Va = norm(V_body);
        
        % 避免奇异点
        if Va > 0.1 
            alpha_a = atan2(w, u);  
            beta_a  = asin(v / Va);   
        else
            alpha_a = 0; beta_a = 0;
        end
        
        Q_dyn = 0.5 * rho_air * Va^2; %动压
        
        % 操纵面差分与共模解析
        del_f_sym  = (Aileron(1) + Aileron(2)) / 2; %共模:左右舵面同向偏转，改变翼型弯度
        del_f_diff = Aileron(1) - Aileron(2);      
        del_r_sym  = (Aileron(3) + Aileron(4)) / 2;  
        del_r_diff = Aileron(3) - Aileron(4);       

        % A. 前翼
        CL_f = Aero.CL0Front + Aero.CLAlphaFront * alpha_a + Aero.CLAileronFront * del_f_sym;
        CD_f = Aero.CD0Front + Aero.KDFront * CL_f^2;
        Cm_f = Aero.Cm0Front + Aero.CmAileronFront * del_f_sym;
        
        L_f = Q_dyn * Aircraft.AreaWingFront * CL_f;
        D_f = Q_dyn * Aircraft.AreaWingFront * CD_f;
        
        ca = cos(alpha_a); sa = sin(alpha_a);
        F_f_b = [
            -D_f * ca + L_f * sa;
            Q_dyn * Aircraft.AreaWingFront * Aero.CYBetaFront * beta_a;
            -D_f * sa - L_f * ca
        ];
        
        PosAC_f_mean = (Aircraft.PosACWingFrontLeft + Aircraft.PosACWingFrontRight)' / 2; 
        M_f_b = cross(PosAC_f_mean, F_f_b);
        M_f_b(1) = M_f_b(1) + Q_dyn * Aircraft.AreaWingFront * Aircraft.Span * (Aero.ClBetaFront * beta_a + 0.5 * Aero.CLAileronFront * del_f_diff);
        M_f_b(2) = M_f_b(2) + Q_dyn * Aircraft.AreaWingFront * Aircraft.ChordMean * Cm_f;
        M_f_b(3) = M_f_b(3) + Q_dyn * Aircraft.AreaWingFront * Aircraft.Span * Aero.CnBetaFront * beta_a;

        % B. 后翼 (包含下洗干扰)
        eps_wash = Aero.Epsilon0 + Aero.DepsDalpha * alpha_a;
        alpha_r = alpha_a - eps_wash; 
        
        CL_r = Aero.CL0Rear + Aero.CLAlphaRear * alpha_r + Aero.CLAileronRear * del_r_sym;
        CD_r = Aero.CD0Rear + Aero.KDRear * CL_r^2;
        Cm_r = Aero.Cm0Rear + Aero.CmAileronRear * del_r_sym;
        
        L_r = Q_dyn * Aircraft.AreaWingRear * CL_r;
        D_r = Q_dyn * Aircraft.AreaWingRear * CD_r;
        
        ca_r = cos(alpha_r); sa_r = sin(alpha_r);
        F_r_b = [
            -D_r * ca_r + L_r * sa_r;
            Q_dyn * Aircraft.AreaWingRear * Aero.CYBetaRear * beta_a;
            -D_r * sa_r - L_r * ca_r
        ];
        
        PosAC_r_mean = (Aircraft.PosACWingRearLeft + Aircraft.PosACWingRearRight)' / 2;
        M_r_b = cross(PosAC_r_mean, F_r_b);
        M_r_b(1) = M_r_b(1) + Q_dyn * Aircraft.AreaWingRear * Aircraft.Span * (Aero.ClBetaRear * beta_a + 0.5 * Aero.CLAileronRear * del_r_diff);
        M_r_b(2) = M_r_b(2) + Q_dyn * Aircraft.AreaWingRear * Aircraft.ChordMean * Cm_r;
        M_r_b(3) = M_r_b(3) + Q_dyn * Aircraft.AreaWingRear * Aircraft.Span * Aero.CnBetaRear * beta_a;

        % C. 汇总气动输出
        F_a_b = F_f_b + F_r_b;
        M_a_b = M_f_b + M_r_b;
    end
end

== matlab function test_8m_0508/速度控制/混控矩阵-带舵面 ==
  settings: updateMethod=DISCRETE
  data: g input; thrust_acc input; motor_pwm output; surface_cmd output; debug41 output; moments input; StructAircraft parameter
function [motor_pwm, surface_cmd, debug41] = fcn(g, thrust_acc, moments, StructAircraft)

    m = StructAircraft.m;
    %mix_mat = StructAircraft.mix_mat;     % 8x3（roll pitch yaw）→ yaw不用了
    %B_surface = StructAircraft.B_surface; % 4x1（yaw分配矩阵）
    % A_motor = StructAircraft.A_motor;
    B_motor = StructAircraft.B_motor;
    % A_surface = StructAircraft.A_surface;
    B_surface = StructAircraft.B_surface;

    LIMIT_MAX = 0.95;
    LIMIT_MIN = 0.0;

    roll_m  = moments(1);
    pitch_m = moments(2); 
    yaw_m   = moments(3);

    %% ==========================================================
    % 1️⃣ 电机：只负责 thrust + roll + pitch
    % ==========================================================

    % 油门反算
    fN_need = thrust_acc*m;
    temp = fN_need/9.8;
    poly_a = 50;  % 二次项系数 (主要贡献)
    poly_b = 3.087;  % 一次项系数
    delta = poly_b^2 + 4 * poly_a * temp/8;
    hover_throttle = (-poly_b + sqrt(delta)) / (2 * poly_a);

    thrust_acc_throttle = hover_throttle * ones(8,1);

    % RP混控（⚠️ 不再包含yaw）
    mix_rp = B_motor(:,1)*roll_m + B_motor(:,2)*pitch_m;

    % 权重
    T_weights = abs(B_motor(:,1)) + abs(B_motor(:,2));
    T_weights = T_weights / max(T_weights + 1e-6);

    %% ==========================================================
    % 2️⃣ RP优先缩放（保留你原逻辑）
    % ==========================================================

    k_rp = 1.0;
    for i = 1:8
        for j = 1:8
            diff_rp_norm = mix_rp(i)/T_weights(i) - mix_rp(j)/T_weights(j);
            if diff_rp_norm > 1e-6
                allowable = LIMIT_MAX/T_weights(j) - LIMIT_MIN/T_weights(i);
                k_rp = min(k_rp, allowable / diff_rp_norm);
            end
        end
    end

    mix_rp_scaled = mix_rp * k_rp;

    %% ==========================================================
    % 3️⃣ Throttle Shift（PX4 Airmode思想）
    % ==========================================================

    shift_req_up   = (LIMIT_MIN - thrust_acc_throttle - mix_rp_scaled) ./ T_weights;
    shift_req_down = (LIMIT_MAX - thrust_acc_throttle - mix_rp_scaled) ./ T_weights;

    min_delta_t = max(shift_req_up);
    max_delta_t = min(shift_req_down);

    delta_t = 0;
    if delta_t < min_delta_t
        delta_t = min_delta_t;
    elseif delta_t > max_delta_t
        delta_t = max_delta_t;
    end

    motor_out = thrust_acc_throttle + delta_t .* T_weights + mix_rp_scaled;

    %% ==========================================================
    % 🚨 关键变化：这里结束电机分配（没有yaw）
    % ==========================================================

    motor_pwm = motor_out;

    %% ==========================================================
    % 4️⃣ 舵面：单独做 yaw（PX4 Control Allocation思想）
    % ==========================================================

    surface_raw = B_surface(:,3)* -yaw_m;   % 4x1   注意舵面是增大偏转角，升力减小

    SURF_MAX = 1.0;
    SURF_MIN = -1.0;

    % ===== PX4式 yaw 限幅（从电机转移到舵面）=====
    k_surface = 1.0;

    for i = 1:4
        if surface_raw(i) > 1e-6
            k_surface = min(k_surface, SURF_MAX / surface_raw(i));
        elseif surface_raw(i) < -1e-6
            k_surface = min(k_surface, abs(SURF_MIN / surface_raw(i)));
        end
    end

    surface_cmd = surface_raw * k_surface;

    %% debug
    debug41 = surface_cmd;

end

== matlab function test_8m_0508/速度控制/角度环 ==
  data: q_sp input; rate_sp output size=3*1; q_curr input; UAV parameter
function rate_sp = fcn_att_control(q_sp, q_curr, UAV)
    % --- 3. 姿态环 (Attitude Loop) ---
    % 输入:
    %   q_sp:     期望四元数
    %   q_curr:   当前四元数 (来自传感器/估算器)
    %   UAV:   包含 UAV.P_att (通常为 [6; 6; 2.8])
    % 输出:
    %   rate_sp:  期望角速率 [p, q, r] (rad/s)


%     UAV.P_att = [1; 1; 1;];

    % 1. 计算逆 (共轭)
    q_curr_inv = [q_curr(1); -q_curr(2); -q_curr(3); -q_curr(4)];
    
    % 2. 误差四元数 q_err = q_sp * q_curr_inv
    % (这里为了简洁省略了四元数乘法展开，实际需手写或用 block)
    % 假设 quatmultiply 函数可用，或者参考我之前的代码手写展开
%     q_err = quat_multiply_custom(q_sp, q_curr_inv);
    q_err = quat_multiply_custom(q_curr_inv, q_sp);
    
    % 3. 符号检查 (Double Cover)
    if q_err(1) < 0
        q_err = -q_err;
    end
    
    % 4. 提取虚部并应用 P 增益
    % PX4逻辑: rate_sp = gain * (2 * q_err_imaginary)
    % 乘以2是因为小角度下 2*sin(theta/2) approx theta
    rate_sp = zeros(3,1);
    rate_sp(1) = UAV.P_att(1) * (2 * q_err(2)); % Roll
    rate_sp(2) = UAV.P_att(2) * (2 * q_err(3)); % Pitch
    rate_sp(3) = UAV.P_att(3) * (2 * q_err(4)); % Yaw
    
    % 5. 角速度限幅 (保护措施)
    MAX_RATE = 220 * (pi/180); % 例如 220 deg/s
    rate_sp(2) = max(min(rate_sp(2), MAX_RATE), -MAX_RATE);
    MAX_RATE = 10 * (pi/180);
    rate_sp(3) = max(min(rate_sp(3), MAX_RATE), -MAX_RATE);
end

function q_out = quat_multiply_custom(q, r)
    % 标准四元数乘法
    q_out = [r(1)*q(1)-r(2)*q(2)-r(3)*q(3)-r(4)*q(4);
             r(1)*q(2)+r(2)*q(1)-r(3)*q(4)+r(4)*q(3);
             r(1)*q(3)+r(2)*q(4)+r(3)*q(1)-r(4)*q(2);
             r(1)*q(4)-r(2)*q(3)+r(3)*q(2)+r(4)*q(1)];
end

== matlab function test_8m_0508/MATLAB Function1 ==
  settings: updateMethod=DISCRETE
  data: vb input; landed_state output; thrust input; dt input; debug output
function [landed_state, debug]  = px4_land_detector_logic(vb, thrust, dt)
% PX4_LAND_DETECTOR_LOGIC 模拟PX4多旋翼触底检测逻辑
%
% 输入:
%   vel_z    - 垂直速度 (m/s, 向上为正)
%   vel_xy   - 水平速度矢量模长 (m/s)
%   thrust   - 当前推力输出 (0.0 ~ 1.0)
%   dt       - 采样周期/步长 (s)
%
% 输出:
%   landed_state - 0: Flying, 1: Maybe Landed, 2: Landed
%   stats        - 包含内部计时器状态的结构体

    %% 1. 配置参数 (可根据实际机型调整)
    persistent timer;
    if isempty(timer)
        timer = 0; % 初始化持久化计时器
    end
    vel_z = vb(3);
    vel_xy = vb(1);
    % 判定阈值
    PARAM_LNDMC_Z_VEL_MAX  = 0.1;   % 垂直速度阈值
    PARAM_LNDMC_XY_VEL_MAX = 990.8;   % 水平速度阈值
    PARAM_MPC_THR_MIN      = 0.1;  % 最小推力阈值 (需根据Tilt-Body怠速调整)
    PARAM_LNDMC_TRIG_TIME  = 1.0;   % 确认着陆所需的持续时间 (s)
    MAYBE_LAND_THR         = 0.25;  % 判定 Maybe Landed 的较短时间阈值

    %% 2. 判定条件 (Condition Logic)
    % 条件1: 垂直速度足够小 (接近0)
    cond_vel_z = abs(vel_z) < PARAM_LNDMC_Z_VEL_MAX;
    
    % 条件2: 水平速度足够小
    cond_vel_xy = abs(vel_xy) < PARAM_LNDMC_XY_VEL_MAX;
    
    % 条件3: 推力接近最低限度 (认为飞行器不再试图维持高度)
    % 实际PX4中会根据加速度计判断是否有地面支撑力，此处简化为推力判定
    %cond_thrust = thrust < (PARAM_MPC_THR_MIN + 0.05);
    cond_thrust = thrust(3) > -1e-2 ;


    %% 3. 状态机逻辑 (State Machine)
    if cond_vel_z && cond_vel_xy && cond_thrust
        % 所有条件满足，计时器累加
        timer = timer + dt;
    else
        % 任何一个条件破坏，计时器重置
        timer = 0;
    end

    % 根据计时器确定状态
    if timer >= PARAM_LNDMC_TRIG_TIME
        landed_state = 2; % LANDED
    elseif timer >= MAYBE_LAND_THR
        landed_state = 1; % MAYBE_LANDED
    else
        landed_state = 0; % FLYING
    end
    debug = [cond_vel_z;cond_vel_xy;cond_thrust];
end

== matlab function test_8m_0508/速度控制/Alt2q1/XYZ-ZYX ==
  data: u input; y output
function y = fcn(u)
    TEMP =  u;
    y = [TEMP(3);TEMP(2);TEMP(1)];
end
